simulink model "ROPOD_Control_incFlockControl"  (R2017b)
settings: Solver=ode1  StartTime=0.0  StopTime=inf  FixedStep=Ts  RelTol=1e-3  EnableMultiTasking=on
PreLoadFcn:
  | init_model
InitFcn:
  | init_model
values from neighbouring files (symbols this model uses):
  AgentNumber = 1    [init_model.m]
  FFtheta_intia = 0    [init_model.m]
  FFxy_mass = 0*80    (= 0)    [init_model.m]
  flock_FFtheta_friction = 50    [init_model.m]
  flock_FFxy_friction = 100    [init_model.m]
  I_fhz_ddelta_cntr = 0    [init_model.m]
  I_fhz_dtheta_cntr = 0.3    [init_model.m]
  I_fhz_dtheta_flock_cntr = 0.1    [init_model.m]
  I_fhz_dvarphi_cntr = 0    [init_model.m]
  I_fhz_dxdy_cntr = 0.25    [init_model.m]
  I_fhz_dxdy_flock_cntr = 0.1    [init_model.m]
  K_gain_ddelta_cntr = 0.1    [init_model.m]
  K_gain_dtheta_cntr = 150    [init_model.m]
  K_gain_dtheta_flock_cntr = 100    [init_model.m]
  K_gain_dvarphi_cntr = 0.05    [init_model.m]
  K_gain_dxdy_cntr = 200    [init_model.m]
  K_gain_dxdy_flock_cntr = 200    [init_model.m]
  LL_wp_fhz_ddelta_cntr = 2    [init_model.m]
  LL_wp_fhz_dtheta_cntr = 20    [init_model.m]
  LL_wp_fhz_dtheta_flock_cntr = 20    [init_model.m]
  LL_wp_fhz_dvarphi_cntr = 10    [init_model.m]
  LL_wp_fhz_dxdy_cntr = 20    [init_model.m]
  LL_wp_fhz_dxdy_flock_cntr = 20    [init_model.m]
  LL_wz_fhz_ddelta_cntr = 2    [init_model.m]
  LL_wz_fhz_dtheta_cntr = 20    [init_model.m]
  LL_wz_fhz_dtheta_flock_cntr = 20    [init_model.m]
  LL_wz_fhz_dvarphi_cntr = 2    [init_model.m]
  LL_wz_fhz_dxdy_cntr = 20    [init_model.m]
  LL_wz_fhz_dxdy_flock_cntr = 20    [init_model.m]
  LPF_fhz_ddelta_cntr = 50    [init_model.m]
  LPF_fhz_ddelta_meas = 50    [init_model.m]
  LPF_fhz_dtheta_cntr = 100    [init_model.m]
  LPF_fhz_dtheta_flock_cntr = 40    [init_model.m]
  LPF_fhz_dvarphi_cntr = 50    [init_model.m]
  LPF_fhz_dvarphi_meas = 50    [init_model.m]
  LPF_fhz_dxdy_cntr = 100    [init_model.m]
  LPF_fhz_dxdy_flock_cntr = 40    [init_model.m]
  max_flock_acc_theta = 0.5    [init_model.m]
  max_flock_acc_xy = 0.5    [init_model.m]
  max_flock_vel_theta = 1.0    (= 1)    [init_model.m]
  max_flock_vel_xy = 1.0    (= 1)    [init_model.m]
  max_hw_tau = 7.0    (= 7)    [init_model.m]
  max_ropod_acc_theta = 1.6    [init_model.m]
  max_ropod_acc_xy = 2.0    (= 2)    [init_model.m]
  max_ropod_sw_force = 500    [init_model.m]
  max_ropod_sw_tau = 250    [init_model.m]
  max_ropod_vel_theta = 1.6    [init_model.m]
  max_ropod_vel_xy = 2.0    (= 2)    [init_model.m]
  max_sw_current = 10    [init_model.m]
  Nagents = 2    [init_model.m]
  Nwheels = 4    [Jqwl_numeric_function.m]    (also in S_matrix.m; extract_kinmodel_parameters.m; init_model.m; tau_optimal_dist_vec_fun.m)
  pivot_offs_sws = [0.0243    0.4689    0.3384    5.9050]    [init_model.m]
  ropod_kinmodel_pv = struct2array(ropod_kinmodel_param)    [set_ropod_KinModparams.m]
  ropod_position_inflock = [-1 0 3.1416]    [init_model.m]
  SW_COM1_ENABLE1 = hex2dec('0001')    [init_model.m]
  SW_COM1_ENABLE2 = hex2dec('0002')    [init_model.m]
  SW_COM1_MODE_TORQUE = bitshift(hex2dec('0000'),2)    [init_model.m]
  SW_COM1_MODE_VELOCITY = bitshift(hex2dec('0002'),2)    [init_model.m]
  SW_COM1_USE_TS = hex2dec('8000')    [init_model.m]
  Tinit = 2    [init_model.m]
  Ts = 0.001    [init_model.m]
  Tsflck = 0.01    [init_model.m]
undefined symbols (not defined in the file or in its folder): DiscIntNeverNeededParam, sw_tau_2_curr
libraries: simulink x78, cstblocks x30, dspsigops x12, SOEM_EtherCAT_Lib x5, dspnetwork x4
(part 1 of 6)
settings Model: SimulationMode=external  Creator=cesar  LastModifiedBy=cesar
settings DataIOCC: SaveFormat=Array  LoggingToFile=on
settings OptimizationCC: DefaultParameterBehavior=Inlined  UseFloatMulNetSlope=on  InlineInvariantSignals=on  PassReuseOutputArgsThreshold=0  EfficientFloat2IntCast=on  MaxStackSize=64
settings DebuggingCC: ParameterTunabilityLossMsg=error  UnderSpecifiedDataTypeMsg=warning  ModelReferenceDataLoggingMessage=error
settings HardwareCC: ProdBitPerLong=64  ProdHWDeviceType=Intel->x86-64 (Linux 64)  TargetBitPerLong=64  TargetBitPerPointer=64  TargetBitPerSizeT=64  TargetBitPerPtrDiffT=64  TargetLargestAtomicFloat=Float  TargetIntDivRoundTo=Zero  TargetEndianess=LittleEndian  TargetWordSize=64  TargetHWDeviceType=Intel->x86-64 (Linux 64)
settings SFSimCC: SFSimEcho=off  MATLABDynamicMemAlloc=off
settings RTWCC: SystemTargetFile=mttarget.tlc  MakeCommand="make_rtw  CC=\"ccache gcc\" OPTS=\"-DNETIF_ID=0 -DTEST_CONN_MODEL -D_GNU_SOURCE -DPRIO=99\""  TemplateMakefile=mt_unix.tmf  Description=Generic Real-Time Target  GenerateReport=on  Toolchain=Catkin  BuildConfiguration=Faster Runs  LaunchReport=on  RTWCompilerOptimization=Custom  RTWCustomCompilerOptimizations=-O2 -g -W
settings RTWCC: CustomInclude=|
  | /usr/local/include/soem
  | gamepad_source_files/
settings RTWCC: CustomSource=|
  | gamepad_source_files/gamepad.c
  | gamepad_source_files/joystick.c
  | gamepad_source_files/joystick_read_sticks_wrapper.c
  | gamepad_source_files/joystick_read_sticks.c
settings RTWCC: CustomLibrary=|
  | /usr/local/lib/libsoem.so
  | /usr/local/MATLAB/R2017b/bin/glnxa64/libmwnetworkdevice.so
  | /usr/lib/x86_64-linux-gnu/libudev.so
settings CodeAppCC: ForceParamTrailComments=on  OperatorAnnotations=on
settings GRTTargetCC: TargetLangStandard=C89/C90 (ANSI)  UseToolchainInfoCompliant=off

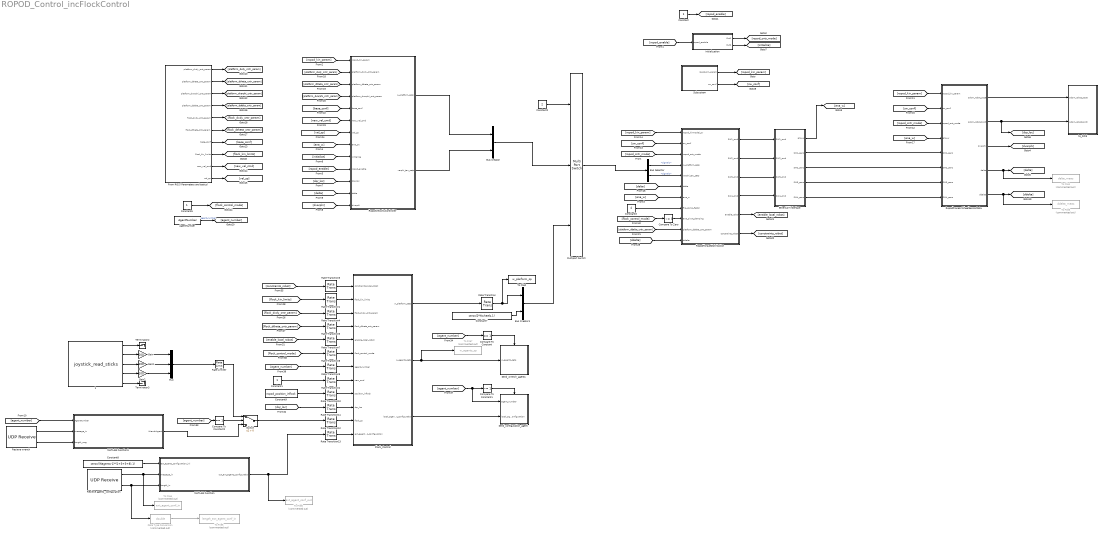
== system ROPOD_Control_incFlockControl ==
  " 1" : S-Function  FunctionName=joystick_read_sticks  SFunctionDeploymentMode=off  EnableBusSupport=off  mask(Legacy Function){SFunctionSpec=double y1 = read_joystick(), ShowSpec=off}
      mask prompts: ShowSpec "Display function specification"
      mask help:
      | This block allows you to call the legacy functions specified by the following Legacy Code Tool definition:
      | def.SFunctionName = 'joystick_read';
      | def.OutputFcnSpec = 'double y1 = read_joystick()';
      | def.StartFcnSpec = 'void init()';
      | def.HeaderFiles = {'joystick.h', 'stdio.h', 'ncurses.h', 'gamepad.h'};
      | def.SourceFiles = {'joystick.c'};
      | def.HostLibFiles = {'libgamepad.so.1'};
      mask Help: <p>This block was generated automatically by the Legacy Code Tool. For detailed help on this tool, call<a href="matlab:legacy_code('help')"> legacy_code('help')</a>.</p>
      mask Callback ShowSpec:
      | if strcmp(get_param(gcbh, 'ShowSpec'), 'on')
      |   set_param(gcbh, 'MaskDisplay', sprintf('fprintf(''%s'');', get_param(gcbh, 'SFunctionSpec')));
      | else
      |   set_param(gcbh, 'MaskDisplay', sprintf('fprintf(''%s'');', get_param(gcbh, 'FunctionName')));
      | end
      mask Display: fprintf('joystick_read_sticks');
  AgentNumber : Constant  Value=AgentNumber
  Bus Creator : BusCreator  Inputs=2
  Bus Creator1 : BusCreator  Inputs=2
  Bus Selector : BusSelector  OutputSignals=signal1,signal2
  Compare To Constant : simulink/Logic and Bit Operations/Compare To Constant  relop===  const=1  OutDataTypeStr=boolean
  Compare To Constant1 : simulink/Logic and Bit Operations/Compare To Constant  relop=~=  const=1  OutDataTypeStr=boolean
  Compare To Constant2 : simulink/Logic and Bit Operations/Compare To Constant  relop===  const=1  OutDataTypeStr=boolean
  Compare To Zero : simulink/Logic and Bit Operations/Compare To Zero  relop=~=  OutDataTypeStr=boolean
  Constant : Constant
  Constant1 : Constant
  Constant2 : Constant  Value=2
  Constant3 : Constant  Value=4
  Constant5 : Constant
  Constant7 : Constant  Value=zeros(2*Nwheels,1)
  Constant8 : Constant  Value=zeros((Nagents-1)*(1+3+3+8),1)
  Constant9 : Constant  Value=ropod_position_inflock
  Data Type Conversion : DataTypeConversion  Commented=on  OutDataTypeStr=double
  EtherCAT Interface : Subsystem
  Flock_Control : Subsystem
  From ROS (Parameters and topics) : Subsystem
  Gain : Gain  Gain=200
  Gain1 : Gain  Gain=200
  Gain2 : Gain  Gain=100
  Initialization : Subsystem
  MATLAB Function : MATLAB Function  TreatAsAtomicUnit=on
  MATLAB Function1 : MATLAB Function  TreatAsAtomicUnit=on
  Multiport Switch : MultiPortSwitch  Inputs=2
  Mux : Mux  Inputs=3
  Rate Limiter : RateLimiter  RisingSlewLimit=200  FallingSlewLimit=-200  SampleTimeMode=inherited
  Rate Transition : RateTransition  OutPortSampleTime=Ts
  Rate Transition{1..5,7..13} (12 alike) : RateTransition  OutPortSampleTime=Tsflck
  Recieve agents_configuration : dspnetwork/UDP Receive  localURL='0.0.0.0'  localPort=25002  remoteURL='0.0.0.0'  remotePort=-1  recvBufferSize=8192  dims=(1+1+3+8)  signalDatatype=double  isVarSize=off  showBlockingTime=on  blockingTime=0  sampletime=Ts  blockPlatform=HOST
      settings: SourceProductName=DSP System Toolbox  SourceProductBaseCode=DS
  Recieve wrench : dspnetwork/UDP Receive  localURL='0.0.0.0'  localPort=25001  remoteURL='0.0.0.0'  remotePort=-1  recvBufferSize=8192  dims=3*(Nagents-1)  signalDatatype=double  isVarSize=off  showBlockingTime=on  blockingTime=0  sampletime=Ts  blockPlatform=HOST
      settings: SourceProductName=DSP System Toolbox  SourceProductBaseCode=DS
  RopodProcessWheelSensorData : Subsystem
  RopodTorqueDistribution : Subsystem
  RopodVelocityController : Subsystem
  Send_configuration_agent : Subsystem
  Send_wrench_agents : Subsystem
  Subsystem : Subsystem
  Switch : Switch  Criteria=u2 > Threshold
  Terminator2 : Terminator
  Terminator3 : Terminator
  To File1 : ToFile  Commented=on  Filename=delta_meas  MatrixName=delta_meas
  To File2 : ToFile  Filename=w_plarform_sp  MatrixName=w_plarform_sp
  To File3 : ToFile  Commented=on  Filename=ddelta_meas  MatrixName=ddelta_meas
  To File4 : ToFile  Commented=on  Filename=ext_agent_conf_in  MatrixName=ext_agent_conf_in
  To File5 : ToFile  Commented=on  Filename=length_ext_agent_conf_in  MatrixName=length_ext_agent_conf_in
  To File6 : ToFile  Commented=on  Filename=ext_agent_conf_out  MatrixName=ext_agent_conf_out
  To File7 : ToFile  Commented=on  Filename=w_agents_sp  MatrixName=w_agents_sp
  to_ROS : Subsystem
  wires:
  [ena_w] -> RopodProcessWheelSensorData/4(ena_w)
  Rate Transition3/1 -> Flock_Control/1(constraints_local_robot)
  Constant5/1 -> [flock_control_mode]
  [platform_dvarphi_cntr_param] -> RopodVelocityController/4(platform_dvarphi_cntr_param)
  [agent_number] -> MATLAB Function1/1(AgentNumber)
  [ropod_cntr_mode] -> RopodTorqueDistribution/3(ropod_cntr_mode)
  [initialize] -> RopodVelocityController/9(initialize)
  [dqr_loc] -> Rate Transition11/1
  [ropod_kin_param] -> RopodVelocityController/1(ropod_kin_param)
  AgentNumber/1 -> [agent_number]  "agent_number"
  RopodTorqueDistribution/4(SW4_cmd) -> EtherCAT Interface/4(SW4_cmd)
  [ddelta] -> RopodTorqueDistribution/11(ddelta)
  Constant9/1 -> Rate Transition10/1
  [sw_conf] -> RopodProcessWheelSensorData/2(sw_conf)
  Subsystem/2(sw_conf) -> [sw_conf]
  Rate Transition5/1 -> Flock_Control/4(flock_dtheta_cntr_param)
  From ROS (Parameters and topics)/9(new_vel_cmd) -> [new_vel_cmd]
  [dqr_loc] -> RopodVelocityController/11(dqr_loc)
  [ropod_cntr_mode] -> RopodProcessWheelSensorData/3(ropod_cntr_mode)
  Recieve agents_configuration/1 -> To File4/1, MATLAB Function/2(message_in)
  Constant8/1 -> MATLAB Function/1(ext_agents_configuration_ini)
  Constant3/1 -> RopodTorqueDistribution/8(flip_comp_factor)
  Recieve wrench/1 -> MATLAB Function1/2(message_in)
  RopodProcessWheelSensorData/2(odom_robot_twist) -> to_ROS/2(odom_robot_twist), [dqr_loc]
  [platform_dxdy_cntr_param] -> RopodVelocityController/2(platform_dxdy_cntr_param)
  Initialization/2(Out2) -> [initialize]
  RopodTorqueDistribution/2(SW2_cmd) -> EtherCAT Interface/2(SW2_cmd)
  [platform_dtheta_cntr_param] -> RopodVelocityController/3(platform_dtheta_cntr_param)
  From ROS (Parameters and topics)/7(base_conf) -> [base_conf]
  [ropod_enable] -> Initialization/1(ropod_enable)
  RopodProcessWheelSensorData/3(dvarphi) -> [dvarphi]
  [vel_sp] -> RopodVelocityController/7(vel_sp)
  Compare To Constant/1 -> Send_wrench_agents/Enable
  Recieve agents_configuration/2 -> Data Type Conversion/1, MATLAB Function/3(length_in)
  RopodTorqueDistribution/1(SW1_cmd) -> EtherCAT Interface/1(SW1_cmd)
  From ROS (Parameters and topics)/2(platform_dtheta_cntr_param) -> [platform_dtheta_cntr_param]
  Flock_Control/3(local_agent_configuration) -> Send_configuration_agent/2(local_agent_configuration)
  Constant2/1 -> Multiport Switch/1
  Recieve wrench/2 -> MATLAB Function1/3(length_msg)
  From ROS (Parameters and topics)/3(platform_dvarphi_cntr_param) -> [platform_dvarphi_cntr_param]
  [flock_control_mode] -> Rate Transition8/1
  From ROS (Parameters and topics)/6(flock_dtheta_cntr_param) -> [flock_dtheta_cntr_param]
  [delta] -> RopodVelocityController/12(delta)
  [ena_w] -> RopodTorqueDistribution/7(ena_w)
  [flock_dxdy_cntr_param] -> Rate Transition4/1
  [base_conf] -> RopodVelocityController/5(base_conf)
  [flock_dtheta_cntr_param] -> Rate Transition5/1
  EtherCAT Interface/1(ena_w) -> [ena_w]
  Constant/1 -> [ropod_enable]
  [ropod_enable] -> RopodVelocityController/10(ropod_enable)
  [new_vel_cmd] -> RopodVelocityController/6(new_vel_cmd)
  From ROS (Parameters and topics)/1(platform_dxdy_cntr_param) -> [platform_dxdy_cntr_param]
  [agent_number] -> Rate Transition9/1
  [ropod_kin_param] -> RopodProcessWheelSensorData/1(ropod_kin_param)
  [enable_local_robot] -> Rate Transition7/1
  [ropod_kin_param] -> RopodTorqueDistribution/1(ropod_kinmodel_pv)
  EtherCAT Interface/2(SW1_sens) -> RopodProcessWheelSensorData/5(SW1_sens)
  Flock_Control/1(w_platform_setp) -> Rate Transition/1
  [sw_conf] -> RopodTorqueDistribution/2(sw_conf)
  Rate Transition11/1 -> Flock_Control/10(dqr_loc)
  [dvarphi] -> RopodVelocityController/13(dvarphi)
  [ena_w] -> RopodVelocityController/8(ena_sw)
  RopodProcessWheelSensorData/5(ddelta) -> [ddelta], To File3/1
  Rate Transition12/1 -> Flock_Control/11(flock_sp)
  Rate Transition13/1 -> Flock_Control/12(ext_agents_configuration)
  Compare To Zero/1 -> RopodTorqueDistribution/9(ena_pivot_damping)
  Rate Transition10/1 -> Flock_Control/9(position_inflock)
  From ROS (Parameters and topics)/4(platform_ddelta_cntr_param) -> [platform_ddelta_cntr_param]
  [constraints_robot] -> Rate Transition3/1
  Rate Transition7/1 -> Flock_Control/5(enable_local_robot)
  Subsystem/1(ropod_kin_param) -> [ropod_kin_param]
  Rate Transition9/1 -> Flock_Control/7(agent_number)
  [platform_ddelta_cntr_param] -> RopodTorqueDistribution/10(platform_ddelta_cntr_param)
  EtherCAT Interface/5(SW4_sens) -> RopodProcessWheelSensorData/8(SW4_sens)
  [delta] -> RopodTorqueDistribution/6(delta)
  Rate Transition4/1 -> Flock_Control/3(flock_dxdy_cntr_param)
  Flock_Control/2(w_agents_setp) -> To File7/1, Send_wrench_agents/1(w_agents_setp)
  EtherCAT Interface/4(SW3_sens) -> RopodProcessWheelSensorData/7(SW3_sens)
  RopodProcessWheelSensorData/4(delta) -> [delta], To File1/1
  [agent_number] -> Compare To Constant/1
  RopodProcessWheelSensorData/1(odom_robot_pose) -> to_ROS/1(odom_robot_pose)
  Initialization/1(Out1) -> [ropod_cntr_mode]
  From ROS (Parameters and topics)/10(vel_sp) -> [vel_sp]
  Rate Transition8/1 -> Flock_Control/6(flock_control_mode)
  EtherCAT Interface/3(SW2_sens) -> RopodProcessWheelSensorData/6(SW2_sens)
  Compare To Constant1/1 -> Send_configuration_agent/Enable
  RopodTorqueDistribution/3(SW3_cmd) -> EtherCAT Interface/3(SW3_cmd)
  From ROS (Parameters and topics)/5(flock_dxdy_cntr_param) -> [flock_dxdy_cntr_param]
  [flock_control_mode] -> Compare To Zero/1
  [agent_number] -> Send_configuration_agent/1(agent_number), Compare To Constant1/1
  [agent_number] -> Compare To Constant2/1
  Compare To Constant2/1 -> Switch/2
  Mux/1 -> Rate Limiter/1
  Switch/1 -> Rate Transition12/1
  MATLAB Function/1(out_ext_agents_configuration) -> To File6/1, Rate Transition13/1
  RopodVelocityController/1(w_platform_setp) -> Bus Creator/1
  RopodVelocityController/2(varphi_tau_setp) -> Bus Creator/2
  Rate Transition/1 -> To File2/1, Bus Creator1/1
  Constant7/1 -> Bus Creator1/2
  Bus Creator1/1 -> Multiport Switch/3
  Bus Creator/1 -> Multiport Switch/2
  Multiport Switch/1 -> Bus Selector/1
  Bus Selector/1 -> RopodTorqueDistribution/4(w_platform_setp)  "<signal1>"
  Bus Selector/2 -> RopodTorqueDistribution/5(varphi_tau_setp)  "<signal2>"
  Rate Limiter/1 -> Switch/1
  MATLAB Function1/1(WrenchAgent) -> Switch/3
  Data Type Conversion/1 -> To File5/1
  " 1"/3 -> Gain1/1
  Gain1/1 -> Mux/2
  " 1"/5 -> Terminator3/1
  Gain2/1 -> Mux/3
  Gain/1 -> Mux/1
  " 1"/2 -> Gain/1
  " 1"/4 -> Gain2/1
  " 1"/1 -> Terminator2/1
  From ROS (Parameters and topics)/8(flock_kin_limits) -> [flock_kin_limits]
  [flock_kin_limits] -> Rate Transition1/1
  Rate Transition1/1 -> Flock_Control/2(flock_kin_limits)
  RopodTorqueDistribution/5(enable_robot) -> [enable_local_robot]
  RopodTorqueDistribution/6(constraints_robot) -> [constraints_robot]
  Rate Transition2/1 -> Flock_Control/8(new_cmd)
  Constant1/1 -> Rate Transition2/1

== system ROPOD_Control_incFlockControl/EtherCAT Interface ==
  SW1_cmd : Inport
  SW2_cmd : Inport  Port=2
  SW3_cmd : Inport  Port=3
  SW4_cmd : Inport  Port=4
  Constant : Constant  Value=[1 1 1 1]
  Display1 : Display  Commented=on
  ECAT_Interface : SOEM_EtherCAT_Lib/ECAT_Interface  Priority=0  Commented=on  IFINTERFACE=eth0  TS=Ts
      settings: SourceProductName=SOEM_EtherCAT_Lib
  Gain1 : Gain  Commented=on  OutDataTypeStr=double
  Smart_Wheel_1 : Subsystem
  Smart_Wheel_2 : Subsystem
  Smart_Wheel_3 : Subsystem
  Smart_Wheel_4 : Subsystem
  ena_w : Outport
  SW1_sens : Outport  Port=2
  SW2_sens : Outport  Port=3
  SW3_sens : Outport  Port=4
  SW4_sens : Outport  Port=5
  wires:
  Smart_Wheel_2/1(SW2_sens) -> SW2_sens/1  "SW2_sens"
  Smart_Wheel_3/1(SW3_sens) -> SW3_sens/1  "SW3_sens"
  SW4_cmd/1 -> Smart_Wheel_4/1(SW4_cmd)
  SW2_cmd/1 -> Smart_Wheel_2/1(SW2_cmd)
  SW3_cmd/1 -> Smart_Wheel_3/1(SW3_cmd)
  SW1_cmd/1 -> Smart_Wheel_1/1(SW1_cmd)
  Smart_Wheel_1/1(SW1_sens) -> SW1_sens/1  "SW1_sens"
  Smart_Wheel_4/1(SW4_sens) -> SW4_sens/1  "SW4_sens"
  ECAT_Interface/1 -> Gain1/1
  Gain1/1 -> Display1/1
  Constant/1 -> ena_w/1

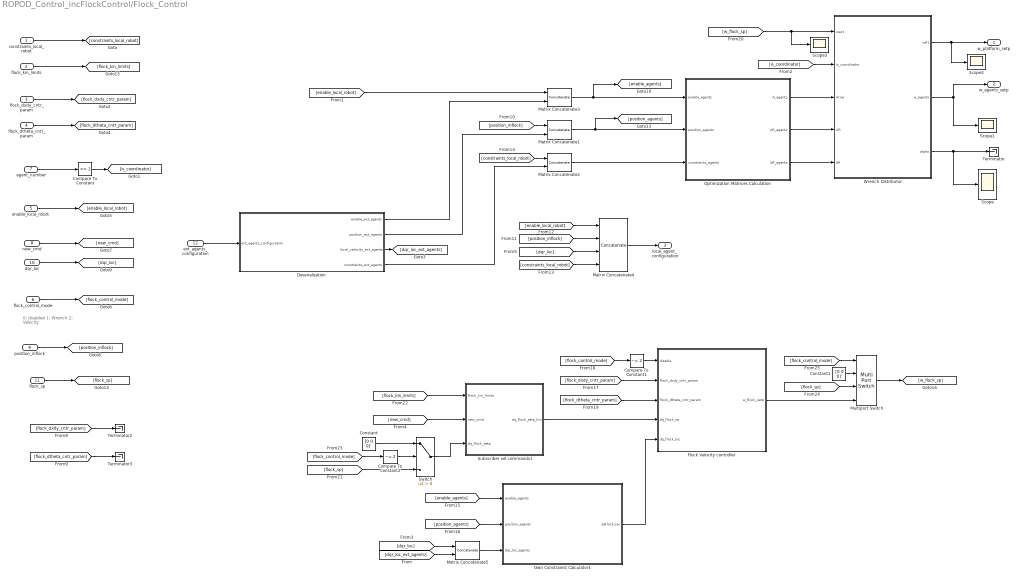
== system ROPOD_Control_incFlockControl/Flock_Control ==
  note: 0: disabled
      | 1: Wrench
      | 2: Velocity
  constraints_local_robot : Inport
  flock_kin_limits : Inport  Port=2
  flock_dxdy_cntr_param : Inport  Port=3
  flock_dtheta_cntr_param : Inport  Port=4
  enable_local_robot : Inport  Port=5
  flock_control_mode : Inport  Port=6
  agent_number : Inport  Port=7
  new_cmd : Inport  Port=8
  position_inflock : Inport  Port=9
  dqr_loc : Inport  Port=10
  flock_sp : Inport  Port=11
  ext_agents_configuration : Inport  Port=12
  Compare To Constant : simulink/Logic and Bit Operations/Compare To Constant  relop===  const=1  OutDataTypeStr=boolean
  Compare To Constant1 : simulink/Logic and Bit Operations/Compare To Constant  relop=~=  const=2  OutDataTypeStr=boolean
  Compare To Constant2 : simulink/Logic and Bit Operations/Compare To Constant  relop=~=  const=2  OutDataTypeStr=boolean
  Constant : Constant  Value=[0 0 0]'
  Constant1 : Constant  Value=[0 0 0]'
  Deserialization : MATLAB Function  TreatAsAtomicUnit=on
  Flock Velocity controller : Subsystem
  Matrix Concatenate1 : Concatenate  Mode=Multidimensional array  ConcatenateDimension=2
  Matrix Concatenate2 : Concatenate  Mode=Multidimensional array  ConcatenateDimension=2
  Matrix Concatenate3 : Concatenate  Mode=Multidimensional array  ConcatenateDimension=2
  Matrix Concatenate4 : Concatenate  NumInputs=4  Mode=Multidimensional array
  Matrix Concatenate5 : Concatenate  Mode=Multidimensional array
  Multiport Switch : MultiPortSwitch  DataPortOrder=Zero-based contiguous
  Optimization Matrices Calculation : MATLAB Function  TreatAsAtomicUnit=on
  Own Constrainst Calculator1 : MATLAB Function  TreatAsAtomicUnit=on
  Scope{,1..3} (4 alike) : Scope
  Subscriber vel commands1 : Subsystem
  Switch : Switch  Criteria=u2 > Threshold
  Terminator : Terminator
  Terminator2 : Terminator
  Terminator3 : Terminator
  Wrench Distributor : MATLAB Function  TreatAsAtomicUnit=on
  w_platform_setp : Outport
  w_agents_setp : Outport  Port=2
  local_agent_configuration : Outport  Port=3
  wires:
  constraints_local_robot/1 -> [constraints_local_robot]
  Wrench Distributor/1(wR1) -> Scope2/1, w_platform_setp/1
  agent_number/1 -> Compare To Constant/1
  [is_coordinator] -> Wrench Distributor/2(is_coordinator)
  Wrench Distributor/2(w_agents) -> Scope1/1, w_agents_setp/1
  Wrench Distributor/3(alpha) -> Scope/1, Terminator/1
  flock_dxdy_cntr_param/1 -> [flock_dxdy_cntr_param]
  flock_dtheta_cntr_param/1 -> [flock_dtheta_cntr_param]
  ext_agents_configuration/1 -> Deserialization/1(ext_agents_configuration)
  Optimization Matrices Calculation/1(A_agents) -> Wrench Distributor/3(Arow)
  Optimization Matrices Calculation/2(AR_agents) -> Wrench Distributor/4(AR)
  Optimization Matrices Calculation/3(bR_agents) -> Wrench Distributor/5(bR)
  Deserialization/1(enable_ext_agents) -> Matrix Concatenate3/2
  Deserialization/4(constraints_ext_agents) -> Matrix Concatenate2/2
  Deserialization/2(position_ext_agents) -> Matrix Concatenate1/2
  Matrix Concatenate2/1 -> Optimization Matrices Calculation/3(constraints_agents)
  Matrix Concatenate1/1 -> [position_agents], Optimization Matrices Calculation/2(position_agents)
  Matrix Concatenate3/1 -> [enable_agents], Optimization Matrices Calculation/1(enable_agents)
  dqr_loc/1 -> [dqr_loc]
  enable_local_robot/1 -> [enable_local_robot]
  [enable_local_robot] -> Matrix Concatenate3/1
  flock_control_mode/1 -> [flock_control_mode]
  [flock_dxdy_cntr_param] -> Terminator2/1
  [flock_dtheta_cntr_param] -> Terminator3/1
  Matrix Concatenate4/1 -> local_agent_configuration/1
  position_inflock/1 -> [position_inflock]
  [position_inflock] -> Matrix Concatenate1/1
  [position_inflock] -> Matrix Concatenate4/2
  Compare To Constant/1 -> [is_coordinator]
  Deserialization/3(local_velocity_ext_agents) -> [dqr_loc_ext_agents]
  [dqr_loc_ext_agents] -> Matrix Concatenate5/2
  [dqr_loc] -> Matrix Concatenate5/1
  Matrix Concatenate5/1 -> Own Constrainst Calculator1/3(dqr_loc_agents)
  [dqr_loc] -> Matrix Concatenate4/3
  [enable_local_robot] -> Matrix Concatenate4/1
  [constraints_local_robot] -> Matrix Concatenate4/4
  [constraints_local_robot] -> Matrix Concatenate2/1
  [position_agents] -> Own Constrainst Calculator1/2(position_agents)
  [enable_agents] -> Own Constrainst Calculator1/1(enable_agents)
  Own Constrainst Calculator1/1(dqflock_loc) -> Flock Velocity controller/5(dq_flock_loc)
  [flock_dxdy_cntr_param] -> Flock Velocity controller/2(flock_dxdy_cntr_param)
  [flock_dtheta_cntr_param] -> Flock Velocity controller/3(flock_dtheta_cntr_param)
  [flock_control_mode] -> Compare To Constant1/1
  Compare To Constant1/1 -> Flock Velocity controller/1(disable)
  [w_flock_sp] -> Scope3/1, Wrench Distributor/1(wact)
  flock_sp/1 -> [flock_sp]
  flock_kin_limits/1 -> [flock_kin_limits]
  [flock_kin_limits] -> Subscriber vel commands1/1(flock_kin_limits)
  Subscriber vel commands1/1(dq_flock_setp_lim) -> Flock Velocity controller/4(dq_flock_sp)
  Compare To Constant2/1 -> Switch/2
  [flock_sp] -> Switch/3
  [flock_control_mode] -> Compare To Constant2/1
  Constant/1 -> Switch/1
  [flock_sp] -> Multiport Switch/3
  [flock_control_mode] -> Multiport Switch/1
  Constant1/1 -> Multiport Switch/2
  Flock Velocity controller/1(w_flock_setp) -> Multiport Switch/4
  Multiport Switch/1 -> [w_flock_sp]
  Switch/1 -> Subscriber vel commands1/3(dq_flock_setp)
  new_cmd/1 -> [new_cmd]
  [new_cmd] -> Subscriber vel commands1/2(new_cmd)

== system ROPOD_Control_incFlockControl/From ROS (Parameters and topics) ==
  note: doing the transformation with the angle from odometry data helps
      | to keep the robot better align during the Identification, especially because
      | we do not have any absolute reference
  Constant1 : Constant
  Controllers conf : Subsystem
  From Workspace1 : FromWorkspace  VariableName=qrefdot  SampleTime=Ts
  Gain1 : Gain
  ROS base conf : Subsystem
  Selector1 : Selector  InputPortWidth=3  IndexOptions=Index vector (dialog)  Indices=3  OutputSizes=1
  flock kin limits : Subsystem
  rot_matrix2 : MATLAB Function  TreatAsAtomicUnit=on
  platform_dxdy_cntr_param : Outport
  platform_dtheta_cntr_param : Outport  Port=2
  platform_dvarphi_cntr_param : Outport  Port=3
  platform_ddelta_cntr_param : Outport  Port=4
  flock_dxdy_cntr_param : Outport  Port=5
  flock_dtheta_cntr_param : Outport  Port=6
  base_conf : Outport  Port=7
  flock_kin_limits : Outport  Port=8
  new_vel_cmd : Outport  Port=9
  vel_sp : Outport  Port=10
  wires:
  Controllers conf/1(platform_dxdy_cntr_param) -> platform_dxdy_cntr_param/1
  Constant1/1 -> new_vel_cmd/1
  Gain1/1 -> vel_sp/1
  ROS base conf/1(base_conf) -> base_conf/1
  From Workspace1/1 -> Selector1/1, rot_matrix2/1(dqr_glb)
  Controllers conf/3(platform_dvarphi_cntr_param) -> platform_dvarphi_cntr_param/1
  Controllers conf/2(platform_dtheta_cntr_param) -> platform_dtheta_cntr_param/1
  Selector1/1 -> rot_matrix2/2(theta)
  rot_matrix2/1(dqr_loc) -> Gain1/1
  Controllers conf/4(platform_ddelta_cntr_param) -> platform_ddelta_cntr_param/1
  Controllers conf/5(flock_dxdy_cntr_param) -> flock_dxdy_cntr_param/1
  Controllers conf/6(flock_dtheta_cntr_param) -> flock_dtheta_cntr_param/1
  flock kin limits/1(flock_kin_limits) -> flock_kin_limits/1

== system ROPOD_Control_incFlockControl/Initialization ==
  ropod_enable : Inport
  Allow Tinit seconds for initialization : simulink/Logic and Bit Operations/Compare To Constant  relop=<  const=Tinit  OutDataTypeStr=boolean
  Constant : Constant  Value=2
  Constant1 : Constant
  Constant2 : Constant  Value=0
  Digital Clock : DigitalClock  SampleTime=Ts
  Gain : Gain
  Gain1 : Gain  OutDataTypeStr=double
  Switch : Switch  Criteria=u2 > Threshold
  Switch1 : Switch  Criteria=u2 > Threshold
  Out1 : Outport
  Out2 : Outport  Port=2
  wires:
  Switch/1 -> Switch1/1
  Constant1/1 -> Switch/3
  Switch1/1 -> Gain/1
  Digital Clock/1 -> Allow Tinit seconds for initialization/1
  Allow Tinit seconds for initialization/1 -> Gain1/1, Switch/2
  Constant2/1 -> Switch1/3
  Constant/1 -> Switch/1
  ropod_enable/1 -> Switch1/2
  Gain/1 -> Out1/1
  Gain1/1 -> Out2/1

== system ROPOD_Control_incFlockControl/RopodProcessWheelSensorData ==
  ropod_kin_param : Inport
  sw_conf : Inport  Port=2
  ropod_cntr_mode : Inport  Port=3
  ena_w : Inport  Port=4
  SW1_sens : Inport  Port=5
  SW2_sens : Inport  Port=6
  SW3_sens : Inport  Port=7
  SW4_sens : Inport  Port=8
  Compare To Constant : simulink/Logic and Bit Operations/Compare To Constant  relop=~=  const=1  OutDataTypeStr=boolean
  Odometry and Measurement model 4SW : Subsystem
  ROPOD_4Wheel_sens : Subsystem
  odom_robot_pose : Outport
  odom_robot_twist : Outport  Port=2
  dvarphi : Outport  Port=3
  delta : Outport  Port=4
  ddelta : Outport  Port=5
  wires:
  ropod_kin_param/1 -> Odometry and Measurement model 4SW/1(param_in)
  Odometry and Measurement model 4SW/2(odom_robot_twist) -> odom_robot_twist/1
  SW2_sens/1 -> ROPOD_4Wheel_sens/4(SW2_sens)
  ROPOD_4Wheel_sens/3(ddelta) -> ddelta/1
  Odometry and Measurement model 4SW/1(odom_robot_pose) -> odom_robot_pose/1
  ROPOD_4Wheel_sens/2(delta) -> Odometry and Measurement model 4SW/4(delta), delta/1
  SW4_sens/1 -> ROPOD_4Wheel_sens/6(SW4_sens)
  ROPOD_4Wheel_sens/1(dvarphi) -> Odometry and Measurement model 4SW/3(dvarphi), dvarphi/1
  SW3_sens/1 -> ROPOD_4Wheel_sens/5(SW3_sens)
  SW1_sens/1 -> ROPOD_4Wheel_sens/3(SW1_sens)
  Compare To Constant/1 -> ROPOD_4Wheel_sens/1(disable)
  sw_conf/1 -> ROPOD_4Wheel_sens/2(sw_conf)
  ropod_cntr_mode/1 -> Compare To Constant/1
  ena_w/1 -> Odometry and Measurement model 4SW/2(ena_w)

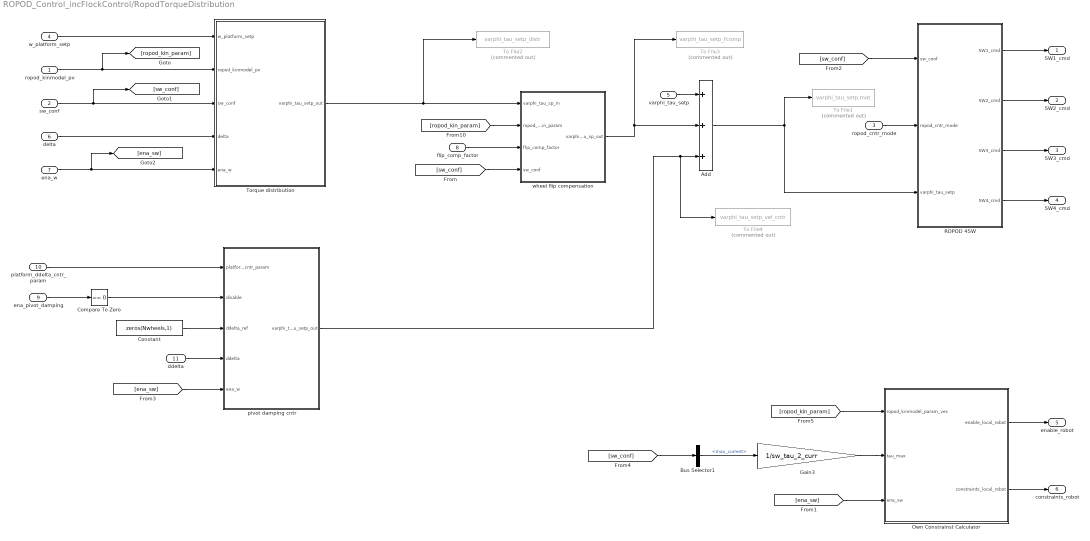
== system ROPOD_Control_incFlockControl/RopodTorqueDistribution ==
  ropod_kinmodel_pv : Inport
  sw_conf : Inport  Port=2
  ropod_cntr_mode : Inport  Port=3
  w_platform_setp : Inport  Port=4
  varphi_tau_setp : Inport  Port=5
  delta : Inport  Port=6
  ena_w : Inport  Port=7
  flip_comp_factor : Inport  Port=8
  ena_pivot_damping : Inport  Port=9
  platform_ddelta_cntr_param : Inport  Port=10
  ddelta : Inport  Port=11
  Add : Sum  Inputs=+++
  Bus Selector1 : BusSelector  OutputSignals=max_current
  Compare To Zero : simulink/Logic and Bit Operations/Compare To Zero  relop===  OutDataTypeStr=boolean
  Constant : Constant  Value=zeros(Nwheels,1)
  Gain3 : Gain  Gain=1/sw_tau_2_curr
  Own Constrainst Calculator : MATLAB Function  TreatAsAtomicUnit=on
  ROPOD 4SW : Subsystem
  To File1 : ToFile  Commented=on  Filename=varphi_tau_setp.mat  MatrixName=varphi_tau_setp
  To File2 : ToFile  Commented=on  Filename=varphi_tau_setp_distr  MatrixName=varphi_tau_setp_distr
  To File3 : ToFile  Commented=on  Filename=varphi_tau_setp_fcomp  MatrixName=varphi_tau_setp_fcomp
  To File4 : ToFile  Commented=on  Filename=varphi_tau_setp_vel_cntr  MatrixName=varphi_tau_setp_vel_cntr
  Torque distribution : Subsystem
  pivot damping cntr : Subsystem
  wheel flip compensation : Subsystem
  SW1_cmd : Outport
  SW2_cmd : Outport  Port=2
  SW3_cmd : Outport  Port=3
  SW4_cmd : Outport  Port=4
  enable_robot : Outport  Port=5
  constraints_robot : Outport  Port=6
  wires:
  ROPOD 4SW/4(SW4_cmd) -> SW4_cmd/1
  w_platform_setp/1 -> Torque distribution/1(w_platform_setp)
  ropod_kinmodel_pv/1 -> [ropod_kin_param], Torque distribution/2(ropod_kinmodel_pv)
  Add/1 -> To File1/1, ROPOD 4SW/3(varphi_tau_setp)
  ROPOD 4SW/1(SW1_cmd) -> SW1_cmd/1
  ena_w/1 -> [ena_sw], Torque distribution/5(ena_w)
  ROPOD 4SW/3(SW3_cmd) -> SW3_cmd/1
  ropod_cntr_mode/1 -> ROPOD 4SW/2(ropod_cntr_mode)
  [sw_conf] -> ROPOD 4SW/1(sw_conf)
  ROPOD 4SW/2(SW2_cmd) -> SW2_cmd/1
  varphi_tau_setp/1 -> Add/1
  sw_conf/1 -> [sw_conf], Torque distribution/3(sw_conf)
  delta/1 -> Torque distribution/4(delta)
  [ropod_kin_param] -> wheel flip compensation/2(ropod_kin_param)
  wheel flip compensation/1(varphi_tau_sp_out) -> To File3/1, Add/2
  flip_comp_factor/1 -> wheel flip compensation/3(flip_comp_factor)
  Compare To Zero/1 -> pivot damping cntr/2(disable)
  ddelta/1 -> pivot damping cntr/4(ddelta)
  ena_pivot_damping/1 -> Compare To Zero/1
  platform_ddelta_cntr_param/1 -> pivot damping cntr/1(platform_ddelta_cntr_param)
  [ena_sw] -> pivot damping cntr/5(ena_w)
  Constant/1 -> pivot damping cntr/3(ddelta_ref)
  Torque distribution/1(varphi_tau_setp_out) -> To File2/1, wheel flip compensation/1(varphi_tau_sp_in)
  pivot damping cntr/1(varphi_tau_setp_out) -> To File4/1, Add/3
  [sw_conf] -> wheel flip compensation/4(sw_conf)
  [ena_sw] -> Own Constrainst Calculator/3(ena_sw)
  Bus Selector1/1 -> Gain3/1  "<max_current>"
  [sw_conf] -> Bus Selector1/1
  Gain3/1 -> Own Constrainst Calculator/2(tau_max)
  Own Constrainst Calculator/1(enable_local_robot) -> enable_robot/1
  Own Constrainst Calculator/2(constraints_local_robot) -> constraints_robot/1
  [ropod_kin_param] -> Own Constrainst Calculator/1(ropod_kinmodel_param_vec)

== system ROPOD_Control_incFlockControl/RopodVelocityController ==
  ropod_kin_param : Inport
  platform_dxdy_cntr_param : Inport  Port=2
  platform_dtheta_cntr_param : Inport  Port=3
  platform_dvarphi_cntr_param : Inport  Port=4
  base_conf : Inport  Port=5
  new_vel_cmd : Inport  Port=6
  vel_sp : Inport  Port=7
  ena_sw : Inport  Port=8
  initialize : Inport  Port=9
  ropod_enable : Inport  Port=10
  dqr_loc : Inport  Port=11
  delta : Inport  Port=12
  dvarphi : Inport  Port=13
  Logical Operator : Logic  Operator=OR  AllPortsSameDT=off  OutDataTypeStr=boolean
  Logical Operator1 : Logic  Operator=NOT  AllPortsSameDT=off  OutDataTypeStr=boolean
  Subscriber vel commands1 : Subsystem
  platform vel cntr : Subsystem
  w_platform_setp : Outport
  varphi_tau_setp : Outport  Port=2
  wires:
  platform_dvarphi_cntr_param/1 -> [platform_dvarphi_cntr_param]
  platform_dxdy_cntr_param/1 -> [platform_dxdy_cntr_param]
  ropod_kin_param/1 -> [ropod_kin_param]
  platform_dtheta_cntr_param/1 -> [platform_dtheta_cntr_param]
  [ropod_kin_param] -> platform vel cntr/1(ropod_kinmodel_pv)
  vel_sp/1 -> Subscriber vel commands1/3(dq_setp)
  Subscriber vel commands1/1(dq_loc) -> platform vel cntr/6(dqr_sp)
  base_conf/1 -> Subscriber vel commands1/1(base_conf)
  ena_sw/1 -> platform vel cntr/9(ena_w)
  new_vel_cmd/1 -> Subscriber vel commands1/2(new_cmd)
  [platform_dtheta_cntr_param] -> platform vel cntr/4(platform_dtheta_cntr_param)
  [platform_dxdy_cntr_param] -> platform vel cntr/3(platform_dxdy_cntr_param)
  [platform_dvarphi_cntr_param] -> platform vel cntr/5(platform_dxdy_cntr_param1)
  dqr_loc/1 -> platform vel cntr/7(dqr_loc)
  delta/1 -> platform vel cntr/8(delta)
  dvarphi/1 -> platform vel cntr/10(dvarphi)
  platform vel cntr/2(varphi_tau_setp) -> varphi_tau_setp/1
  platform vel cntr/1(w_platform_setp) -> w_platform_setp/1
  ropod_enable/1 -> Logical Operator1/1
  Logical Operator1/1 -> Logical Operator/2
  Logical Operator/1 -> platform vel cntr/2(disable)
  initialize/1 -> Logical Operator/1

== system ROPOD_Control_incFlockControl/Send_configuration_agent ==
  agent_number : Inport
  local_agent_configuration : Inport  Port=2
  Enable : EnablePort
  UDP Send : dspnetwork/UDP Send  remoteURL='255.255.255.255'  remotePort=25002  localURL='0.0.0.0'  localPortSource=Automatically determine  localPort=-1  sampletime=-1  blockPlatform=[]  separateLengthPort=0
      settings: SourceProductName=DSP System Toolbox  SourceProductBaseCode=DS
  Vector Concatenate : Concatenate
  wires:
  agent_number/1 -> Vector Concatenate/1
  local_agent_configuration/1 -> Vector Concatenate/2
  Vector Concatenate/1 -> UDP Send/1

== system ROPOD_Control_incFlockControl/Send_wrench_agents ==
  w_agents_setp : Inport
  Enable : EnablePort
  UDP Send : dspnetwork/UDP Send  remoteURL='255.255.255.255'  remotePort=25001  localURL='0.0.0.0'  localPortSource=Automatically determine  localPort=-1  sampletime=-1  blockPlatform=[]  separateLengthPort=0
      settings: SourceProductName=DSP System Toolbox  SourceProductBaseCode=DS
  wires:
  w_agents_setp/1 -> UDP Send/1

== system ROPOD_Control_incFlockControl/Subsystem ==
  Ropod kinematic parameters : Subsystem
  Smart wheels conf1 : Subsystem
  ropod_kin_param : Outport
  sw_conf : Outport  Port=2
  wires:
  Ropod kinematic parameters/1(ropod_kin_param) -> ropod_kin_param/1
  Smart wheels conf1/1(sw_conf) -> sw_conf/1

== system ROPOD_Control_incFlockControl/to_ROS ==
  odom_robot_pose : Inport
  odom_robot_twist : Inport  Port=2
  Terminator1 : Terminator
  Terminator2 : Terminator
  wires:
  odom_robot_pose/1 -> Terminator2/1
  odom_robot_twist/1 -> Terminator1/1

== system ROPOD_Control_incFlockControl/EtherCAT Interface/Smart_Wheel_1 ==
  SW1_cmd : Inport
  Bus Creator1 : BusCreator  Inputs=40
  Bus Selector : BusSelector  OutputSignals=command1,command2,setpoint1,setpoint2,limit1_p,limit1_n,limit2_p,limit2_n,timestamp
  ec_ROPOD_SmartWheel : SOEM_EtherCAT_Lib/ec_ROPOD_SmartWheel  link_id=1
      settings: SourceProductName=SOEM_EtherCAT_Lib
  SW1_sens : Outport
  wires:
  Bus Creator1/1 -> SW1_sens/1
  ec_ROPOD_SmartWheel/21 -> Bus Creator1/21  "current_2_u"
  ec_ROPOD_SmartWheel/3 -> Bus Creator1/3  "sensor_ts"
  ec_ROPOD_SmartWheel/34 -> Bus Creator1/34  "accel_y"
  ec_ROPOD_SmartWheel/29 -> Bus Creator1/29  "encoder_pivot"
  ec_ROPOD_SmartWheel/18 -> Bus Creator1/18  "velocity_2"
  ec_ROPOD_SmartWheel/19 -> Bus Creator1/19  "current_2_d"
  ec_ROPOD_SmartWheel/14 -> Bus Creator1/14  "voltage_1_v"
  ec_ROPOD_SmartWheel/6 -> Bus Creator1/6  "velocity_1"
  ec_ROPOD_SmartWheel/12 -> Bus Creator1/12  "voltage_1"
  ec_ROPOD_SmartWheel/35 -> Bus Creator1/35  "accel_z"
  ec_ROPOD_SmartWheel/2 -> Bus Creator1/2  "status2"
  ec_ROPOD_SmartWheel/1 -> Bus Creator1/1  "status1"
  ec_ROPOD_SmartWheel/22 -> Bus Creator1/22  "current_2_v"
  ec_ROPOD_SmartWheel/25 -> Bus Creator1/25  "voltage_2_u"
  ec_ROPOD_SmartWheel/24 -> Bus Creator1/24  "voltage_2"
  ec_ROPOD_SmartWheel/15 -> Bus Creator1/15  "voltage_1_w"
  ec_ROPOD_SmartWheel/9 -> Bus Creator1/9  "current_1_u"
  ec_ROPOD_SmartWheel/28 -> Bus Creator1/28  "temperature_2"
  ec_ROPOD_SmartWheel/37 -> Bus Creator1/37  "gyro_y"
  ec_ROPOD_SmartWheel/20 -> Bus Creator1/20  "current_2_q"
  ec_ROPOD_SmartWheel/38 -> Bus Creator1/38  "gyro_z"
  ec_ROPOD_SmartWheel/13 -> Bus Creator1/13  "voltage_1_u"
  ec_ROPOD_SmartWheel/27 -> Bus Creator1/27  "voltage_2_w"
  ec_ROPOD_SmartWheel/7 -> Bus Creator1/7  "current_1_d"
  ec_ROPOD_SmartWheel/5 -> Bus Creator1/5  "encoder_1"
  ec_ROPOD_SmartWheel/36 -> Bus Creator1/36  "gyro_x"
  ec_ROPOD_SmartWheel/23 -> Bus Creator1/23  "current_2_w"
  ec_ROPOD_SmartWheel/4 -> Bus Creator1/4  "setpoint_ts"
  ec_ROPOD_SmartWheel/17 -> Bus Creator1/17  "encoder_2"
  ec_ROPOD_SmartWheel/11 -> Bus Creator1/11  "current_1_w"
  ec_ROPOD_SmartWheel/40 -> Bus Creator1/40  "pressure"
  ec_ROPOD_SmartWheel/30 -> Bus Creator1/30  "velocity_pivot"
  ec_ROPOD_SmartWheel/10 -> Bus Creator1/10  "current_1_v"
  ec_ROPOD_SmartWheel/39 -> Bus Creator1/39  "temperature_imu"
  ec_ROPOD_SmartWheel/16 -> Bus Creator1/16  "temperature_1"
  ec_ROPOD_SmartWheel/33 -> Bus Creator1/33  "accel_x"
  ec_ROPOD_SmartWheel/26 -> Bus Creator1/26  "voltage_2_v"
  ec_ROPOD_SmartWheel/8 -> Bus Creator1/8  "current_1_q"
  ec_ROPOD_SmartWheel/31 -> Bus Creator1/31  "voltage_bus"
  ec_ROPOD_SmartWheel/32 -> Bus Creator1/32  "imu_ts"
  SW1_cmd/1 -> Bus Selector/1
  Bus Selector/1 -> ec_ROPOD_SmartWheel/1  "<command1>"
  Bus Selector/2 -> ec_ROPOD_SmartWheel/2  "<command2>"
  Bus Selector/3 -> ec_ROPOD_SmartWheel/3  "<setpoint1>"
  Bus Selector/4 -> ec_ROPOD_SmartWheel/4  "<setpoint2>"
  Bus Selector/5 -> ec_ROPOD_SmartWheel/5  "<limit1_p>"
  Bus Selector/6 -> ec_ROPOD_SmartWheel/6  "<limit1_n>"
  Bus Selector/7 -> ec_ROPOD_SmartWheel/7  "<limit2_p>"
  Bus Selector/8 -> ec_ROPOD_SmartWheel/8  "<limit2_n>"
  Bus Selector/9 -> ec_ROPOD_SmartWheel/9  "<timestamp>"

== system ROPOD_Control_incFlockControl/EtherCAT Interface/Smart_Wheel_2 ==
  SW2_cmd : Inport
  Bus Creator1 : BusCreator  Inputs=40
  Bus Selector : BusSelector  OutputSignals=command1,command2,setpoint1,setpoint2,limit1_p,limit1_n,limit2_p,limit2_n,timestamp
  ec_ROPOD_SmartWheel : SOEM_EtherCAT_Lib/ec_ROPOD_SmartWheel  link_id=2
      settings: SourceProductName=SOEM_EtherCAT_Lib
  SW2_sens : Outport
  wires:
  Bus Selector/9 -> ec_ROPOD_SmartWheel/9  "<timestamp>"
  Bus Selector/8 -> ec_ROPOD_SmartWheel/8  "<limit2_n>"
  Bus Selector/7 -> ec_ROPOD_SmartWheel/7  "<limit2_p>"
  Bus Selector/6 -> ec_ROPOD_SmartWheel/6  "<limit1_n>"
  Bus Selector/5 -> ec_ROPOD_SmartWheel/5  "<limit1_p>"
  Bus Selector/4 -> ec_ROPOD_SmartWheel/4  "<setpoint2>"
  Bus Selector/3 -> ec_ROPOD_SmartWheel/3  "<setpoint1>"
  Bus Selector/2 -> ec_ROPOD_SmartWheel/2  "<command2>"
  Bus Selector/1 -> ec_ROPOD_SmartWheel/1  "<command1>"
  SW2_cmd/1 -> Bus Selector/1
  ec_ROPOD_SmartWheel/32 -> Bus Creator1/32  "imu_ts"
  ec_ROPOD_SmartWheel/31 -> Bus Creator1/31  "voltage_bus"
  ec_ROPOD_SmartWheel/8 -> Bus Creator1/8  "current_1_q"
  ec_ROPOD_SmartWheel/26 -> Bus Creator1/26  "voltage_2_v"
  ec_ROPOD_SmartWheel/33 -> Bus Creator1/33  "accel_x"
  ec_ROPOD_SmartWheel/16 -> Bus Creator1/16  "temperature_1"
  ec_ROPOD_SmartWheel/39 -> Bus Creator1/39  "temperature_imu"
  ec_ROPOD_SmartWheel/10 -> Bus Creator1/10  "current_1_v"
  ec_ROPOD_SmartWheel/30 -> Bus Creator1/30  "velocity_pivot"
  ec_ROPOD_SmartWheel/40 -> Bus Creator1/40  "pressure"
  ec_ROPOD_SmartWheel/11 -> Bus Creator1/11  "current_1_w"
  ec_ROPOD_SmartWheel/17 -> Bus Creator1/17  "encoder_2"
  ec_ROPOD_SmartWheel/4 -> Bus Creator1/4  "setpoint_ts"
  ec_ROPOD_SmartWheel/23 -> Bus Creator1/23  "current_2_w"
  ec_ROPOD_SmartWheel/36 -> Bus Creator1/36  "gyro_x"
  ec_ROPOD_SmartWheel/5 -> Bus Creator1/5  "encoder_1"
  ec_ROPOD_SmartWheel/7 -> Bus Creator1/7  "current_1_d"
  ec_ROPOD_SmartWheel/27 -> Bus Creator1/27  "voltage_2_w"
  ec_ROPOD_SmartWheel/13 -> Bus Creator1/13  "voltage_1_u"
  ec_ROPOD_SmartWheel/38 -> Bus Creator1/38  "gyro_z"
  ec_ROPOD_SmartWheel/20 -> Bus Creator1/20  "current_2_q"
  ec_ROPOD_SmartWheel/37 -> Bus Creator1/37  "gyro_y"
  ec_ROPOD_SmartWheel/28 -> Bus Creator1/28  "temperature_2"
  ec_ROPOD_SmartWheel/9 -> Bus Creator1/9  "current_1_u"
  ec_ROPOD_SmartWheel/15 -> Bus Creator1/15  "voltage_1_w"
  ec_ROPOD_SmartWheel/24 -> Bus Creator1/24  "voltage_2"
  ec_ROPOD_SmartWheel/25 -> Bus Creator1/25  "voltage_2_u"
  ec_ROPOD_SmartWheel/22 -> Bus Creator1/22  "current_2_v"
  ec_ROPOD_SmartWheel/1 -> Bus Creator1/1  "status1"
  ec_ROPOD_SmartWheel/2 -> Bus Creator1/2  "status2"
  ec_ROPOD_SmartWheel/35 -> Bus Creator1/35  "accel_z"
  ec_ROPOD_SmartWheel/12 -> Bus Creator1/12  "voltage_1"
  ec_ROPOD_SmartWheel/6 -> Bus Creator1/6  "velocity_1"
  ec_ROPOD_SmartWheel/14 -> Bus Creator1/14  "voltage_1_v"
  ec_ROPOD_SmartWheel/19 -> Bus Creator1/19  "current_2_d"
  ec_ROPOD_SmartWheel/18 -> Bus Creator1/18  "velocity_2"
  ec_ROPOD_SmartWheel/29 -> Bus Creator1/29  "encoder_pivot"
  ec_ROPOD_SmartWheel/34 -> Bus Creator1/34  "accel_y"
  ec_ROPOD_SmartWheel/3 -> Bus Creator1/3  "sensor_ts"
  ec_ROPOD_SmartWheel/21 -> Bus Creator1/21  "current_2_u"
  Bus Creator1/1 -> SW2_sens/1

== system ROPOD_Control_incFlockControl/EtherCAT Interface/Smart_Wheel_3 ==
  SW3_cmd : Inport
  Bus Creator1 : BusCreator  Inputs=40
  Bus Selector : BusSelector  OutputSignals=command1,command2,setpoint1,setpoint2,limit1_p,limit1_n,limit2_p,limit2_n,timestamp
  ec_ROPOD_SmartWheel : SOEM_EtherCAT_Lib/ec_ROPOD_SmartWheel  link_id=3
      settings: SourceProductName=SOEM_EtherCAT_Lib
  SW3_sens : Outport
  wires:
  Bus Creator1/1 -> SW3_sens/1
  ec_ROPOD_SmartWheel/21 -> Bus Creator1/21  "current_2_u"
  ec_ROPOD_SmartWheel/3 -> Bus Creator1/3  "sensor_ts"
  ec_ROPOD_SmartWheel/34 -> Bus Creator1/34  "accel_y"
  ec_ROPOD_SmartWheel/29 -> Bus Creator1/29  "encoder_pivot"
  ec_ROPOD_SmartWheel/18 -> Bus Creator1/18  "velocity_2"
  ec_ROPOD_SmartWheel/19 -> Bus Creator1/19  "current_2_d"
  ec_ROPOD_SmartWheel/14 -> Bus Creator1/14  "voltage_1_v"
  ec_ROPOD_SmartWheel/6 -> Bus Creator1/6  "velocity_1"
  ec_ROPOD_SmartWheel/12 -> Bus Creator1/12  "voltage_1"
  ec_ROPOD_SmartWheel/35 -> Bus Creator1/35  "accel_z"
  ec_ROPOD_SmartWheel/2 -> Bus Creator1/2  "status2"
  ec_ROPOD_SmartWheel/1 -> Bus Creator1/1  "status1"
  ec_ROPOD_SmartWheel/22 -> Bus Creator1/22  "current_2_v"
  ec_ROPOD_SmartWheel/25 -> Bus Creator1/25  "voltage_2_u"
  ec_ROPOD_SmartWheel/24 -> Bus Creator1/24  "voltage_2"
  ec_ROPOD_SmartWheel/15 -> Bus Creator1/15  "voltage_1_w"
  ec_ROPOD_SmartWheel/9 -> Bus Creator1/9  "current_1_u"
  ec_ROPOD_SmartWheel/28 -> Bus Creator1/28  "temperature_2"
  ec_ROPOD_SmartWheel/37 -> Bus Creator1/37  "gyro_y"
  ec_ROPOD_SmartWheel/20 -> Bus Creator1/20  "current_2_q"
  ec_ROPOD_SmartWheel/38 -> Bus Creator1/38  "gyro_z"
  ec_ROPOD_SmartWheel/13 -> Bus Creator1/13  "voltage_1_u"
  ec_ROPOD_SmartWheel/27 -> Bus Creator1/27  "voltage_2_w"
  ec_ROPOD_SmartWheel/7 -> Bus Creator1/7  "current_1_d"
  ec_ROPOD_SmartWheel/5 -> Bus Creator1/5  "encoder_1"
  ec_ROPOD_SmartWheel/36 -> Bus Creator1/36  "gyro_x"
  ec_ROPOD_SmartWheel/23 -> Bus Creator1/23  "current_2_w"
  ec_ROPOD_SmartWheel/4 -> Bus Creator1/4  "setpoint_ts"
  ec_ROPOD_SmartWheel/17 -> Bus Creator1/17  "encoder_2"
  ec_ROPOD_SmartWheel/11 -> Bus Creator1/11  "current_1_w"
  ec_ROPOD_SmartWheel/40 -> Bus Creator1/40  "pressure"
  ec_ROPOD_SmartWheel/30 -> Bus Creator1/30  "velocity_pivot"
  ec_ROPOD_SmartWheel/10 -> Bus Creator1/10  "current_1_v"
  ec_ROPOD_SmartWheel/39 -> Bus Creator1/39  "temperature_imu"
  ec_ROPOD_SmartWheel/16 -> Bus Creator1/16  "temperature_1"
  ec_ROPOD_SmartWheel/33 -> Bus Creator1/33  "accel_x"
  ec_ROPOD_SmartWheel/26 -> Bus Creator1/26  "voltage_2_v"
  ec_ROPOD_SmartWheel/8 -> Bus Creator1/8  "current_1_q"
  ec_ROPOD_SmartWheel/31 -> Bus Creator1/31  "voltage_bus"
  ec_ROPOD_SmartWheel/32 -> Bus Creator1/32  "imu_ts"
  SW3_cmd/1 -> Bus Selector/1
  Bus Selector/1 -> ec_ROPOD_SmartWheel/1  "<command1>"
  Bus Selector/2 -> ec_ROPOD_SmartWheel/2  "<command2>"
  Bus Selector/3 -> ec_ROPOD_SmartWheel/3  "<setpoint1>"
  Bus Selector/4 -> ec_ROPOD_SmartWheel/4  "<setpoint2>"
  Bus Selector/5 -> ec_ROPOD_SmartWheel/5  "<limit1_p>"
  Bus Selector/6 -> ec_ROPOD_SmartWheel/6  "<limit1_n>"
  Bus Selector/7 -> ec_ROPOD_SmartWheel/7  "<limit2_p>"
  Bus Selector/8 -> ec_ROPOD_SmartWheel/8  "<limit2_n>"
  Bus Selector/9 -> ec_ROPOD_SmartWheel/9  "<timestamp>"

== system ROPOD_Control_incFlockControl/EtherCAT Interface/Smart_Wheel_4 ==
  SW4_cmd : Inport
  Bus Creator1 : BusCreator  Inputs=40
  Bus Selector : BusSelector  OutputSignals=command1,command2,setpoint1,setpoint2,limit1_p,limit1_n,limit2_p,limit2_n,timestamp
  ec_ROPOD_SmartWheel : SOEM_EtherCAT_Lib/ec_ROPOD_SmartWheel  link_id=4
      settings: SourceProductName=SOEM_EtherCAT_Lib
  SW4_sens : Outport
  wires:
  Bus Selector/9 -> ec_ROPOD_SmartWheel/9  "<timestamp>"
  Bus Selector/8 -> ec_ROPOD_SmartWheel/8  "<limit2_n>"
  Bus Selector/7 -> ec_ROPOD_SmartWheel/7  "<limit2_p>"
  Bus Selector/6 -> ec_ROPOD_SmartWheel/6  "<limit1_n>"
  Bus Selector/5 -> ec_ROPOD_SmartWheel/5  "<limit1_p>"
  Bus Selector/4 -> ec_ROPOD_SmartWheel/4  "<setpoint2>"
  Bus Selector/3 -> ec_ROPOD_SmartWheel/3  "<setpoint1>"
  Bus Selector/2 -> ec_ROPOD_SmartWheel/2  "<command2>"
  Bus Selector/1 -> ec_ROPOD_SmartWheel/1  "<command1>"
  SW4_cmd/1 -> Bus Selector/1
  ec_ROPOD_SmartWheel/32 -> Bus Creator1/32  "imu_ts"
  ec_ROPOD_SmartWheel/31 -> Bus Creator1/31  "voltage_bus"
  ec_ROPOD_SmartWheel/8 -> Bus Creator1/8  "current_1_q"
  ec_ROPOD_SmartWheel/26 -> Bus Creator1/26  "voltage_2_v"
  ec_ROPOD_SmartWheel/33 -> Bus Creator1/33  "accel_x"
  ec_ROPOD_SmartWheel/16 -> Bus Creator1/16  "temperature_1"
  ec_ROPOD_SmartWheel/39 -> Bus Creator1/39  "temperature_imu"
  ec_ROPOD_SmartWheel/10 -> Bus Creator1/10  "current_1_v"
  ec_ROPOD_SmartWheel/30 -> Bus Creator1/30  "velocity_pivot"
  ec_ROPOD_SmartWheel/40 -> Bus Creator1/40  "pressure"
  ec_ROPOD_SmartWheel/11 -> Bus Creator1/11  "current_1_w"
  ec_ROPOD_SmartWheel/17 -> Bus Creator1/17  "encoder_2"
  ec_ROPOD_SmartWheel/4 -> Bus Creator1/4  "setpoint_ts"
  ec_ROPOD_SmartWheel/23 -> Bus Creator1/23  "current_2_w"
  ec_ROPOD_SmartWheel/36 -> Bus Creator1/36  "gyro_x"
  ec_ROPOD_SmartWheel/5 -> Bus Creator1/5  "encoder_1"
  ec_ROPOD_SmartWheel/7 -> Bus Creator1/7  "current_1_d"
  ec_ROPOD_SmartWheel/27 -> Bus Creator1/27  "voltage_2_w"
  ec_ROPOD_SmartWheel/13 -> Bus Creator1/13  "voltage_1_u"
  ec_ROPOD_SmartWheel/38 -> Bus Creator1/38  "gyro_z"
  ec_ROPOD_SmartWheel/20 -> Bus Creator1/20  "current_2_q"
  ec_ROPOD_SmartWheel/37 -> Bus Creator1/37  "gyro_y"
  ec_ROPOD_SmartWheel/28 -> Bus Creator1/28  "temperature_2"
  ec_ROPOD_SmartWheel/9 -> Bus Creator1/9  "current_1_u"
  ec_ROPOD_SmartWheel/15 -> Bus Creator1/15  "voltage_1_w"
  ec_ROPOD_SmartWheel/24 -> Bus Creator1/24  "voltage_2"
  ec_ROPOD_SmartWheel/25 -> Bus Creator1/25  "voltage_2_u"
  ec_ROPOD_SmartWheel/22 -> Bus Creator1/22  "current_2_v"
  ec_ROPOD_SmartWheel/1 -> Bus Creator1/1  "status1"
  ec_ROPOD_SmartWheel/2 -> Bus Creator1/2  "status2"
  ec_ROPOD_SmartWheel/35 -> Bus Creator1/35  "accel_z"
  ec_ROPOD_SmartWheel/12 -> Bus Creator1/12  "voltage_1"
  ec_ROPOD_SmartWheel/6 -> Bus Creator1/6  "velocity_1"
  ec_ROPOD_SmartWheel/14 -> Bus Creator1/14  "voltage_1_v"
  ec_ROPOD_SmartWheel/19 -> Bus Creator1/19  "current_2_d"
  ec_ROPOD_SmartWheel/18 -> Bus Creator1/18  "velocity_2"
  ec_ROPOD_SmartWheel/29 -> Bus Creator1/29  "encoder_pivot"
  ec_ROPOD_SmartWheel/34 -> Bus Creator1/34  "accel_y"
  ec_ROPOD_SmartWheel/3 -> Bus Creator1/3  "sensor_ts"
  ec_ROPOD_SmartWheel/21 -> Bus Creator1/21  "current_2_u"
  Bus Creator1/1 -> SW4_sens/1

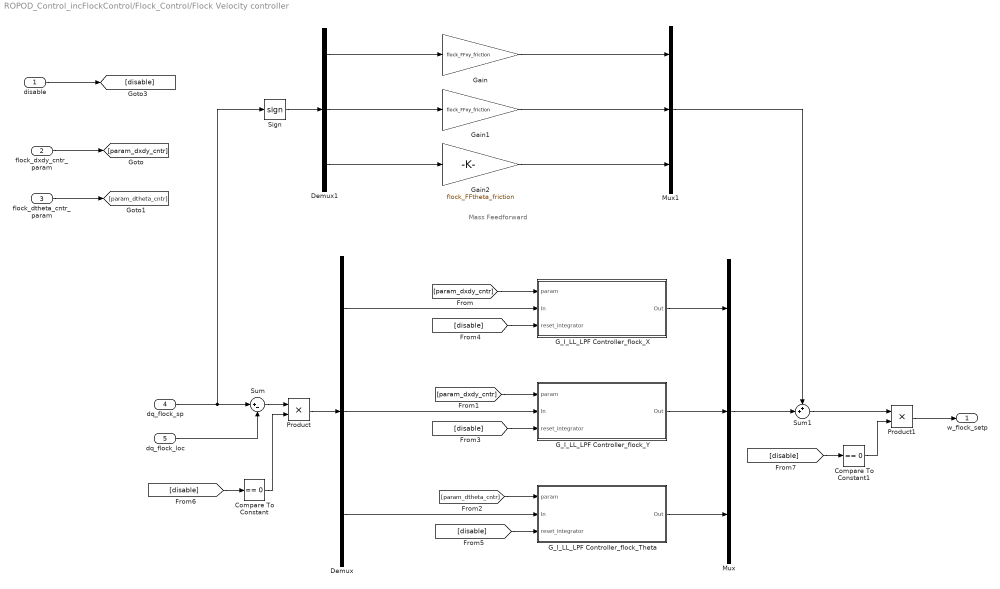
== system ROPOD_Control_incFlockControl/Flock_Control/Flock Velocity controller ==
  note: Mass Feedforward
  disable : Inport
  flock_dxdy_cntr_param : Inport  Port=2
  flock_dtheta_cntr_param : Inport  Port=3
  dq_flock_sp : Inport  Port=4
  dq_flock_loc : Inport  Port=5
  Compare To Constant : simulink/Logic and Bit Operations/Compare To Constant  relop===  const=0  OutDataTypeStr=boolean
  Compare To Constant1 : simulink/Logic and Bit Operations/Compare To Constant  relop===  const=0  OutDataTypeStr=boolean
  Demux : Demux  Outputs=3
  Demux1 : Demux  Outputs=3
  G_I_LL_LPF Controller_flock_Theta : Subsystem
  G_I_LL_LPF Controller_flock_X : Subsystem
  G_I_LL_LPF Controller_flock_Y : Subsystem
  Gain : Gain  Gain=flock_FFxy_friction
  Gain1 : Gain  Gain=flock_FFxy_friction
  Gain2 : Gain  Gain=flock_FFtheta_friction
  Mux : Mux  Inputs=3
  Mux1 : Mux  Inputs=3
  Product : Product
  Product1 : Product
  Sign : Signum
  Sum : Sum  Inputs=|+-
  Sum1 : Sum  Inputs=++|
  w_flock_setp : Outport
  wires:
  G_I_LL_LPF Controller_flock_Theta/1(Out) -> Mux/3
  Demux/1 -> G_I_LL_LPF Controller_flock_X/2(In)
  Demux/2 -> G_I_LL_LPF Controller_flock_Y/2(In)
  G_I_LL_LPF Controller_flock_Y/1(Out) -> Mux/2
  G_I_LL_LPF Controller_flock_X/1(Out) -> Mux/1
  Demux/3 -> G_I_LL_LPF Controller_flock_Theta/2(In)
  dq_flock_sp/1 -> Sign/1, Sum/1
  dq_flock_loc/1 -> Sum/2
  [param_dxdy_cntr] -> G_I_LL_LPF Controller_flock_X/1(param)
  [param_dxdy_cntr] -> G_I_LL_LPF Controller_flock_Y/1(param)
  [param_dtheta_cntr] -> G_I_LL_LPF Controller_flock_Theta/1(param)
  disable/1 -> [disable]
  [disable] -> G_I_LL_LPF Controller_flock_X/3(reset_integrator)
  [disable] -> G_I_LL_LPF Controller_flock_Y/3(reset_integrator)
  flock_dxdy_cntr_param/1 -> [param_dxdy_cntr]
  flock_dtheta_cntr_param/1 -> [param_dtheta_cntr]
  [disable] -> G_I_LL_LPF Controller_flock_Theta/3(reset_integrator)
  Sign/1 -> Demux1/1
  Demux1/1 -> Gain/1
  Gain/1 -> Mux1/1
  Demux1/2 -> Gain1/1
  Gain1/1 -> Mux1/2
  Demux1/3 -> Gain2/1
  Gain2/1 -> Mux1/3
  Mux1/1 -> Sum1/1
  Mux/1 -> Sum1/2
  Sum/1 -> Product/1
  Product/1 -> Demux/1
  Compare To Constant/1 -> Product/2
  [disable] -> Compare To Constant/1
  [disable] -> Compare To Constant1/1
  Sum1/1 -> Product1/1
  Compare To Constant1/1 -> Product1/2
  Product1/1 -> w_flock_setp/1
